simulink model "sudoku"  (R2012b)
settings: Solver=ode45  StartTime=0.0  StopTime=10.0  RelTol=1e-3
libraries: sldvlib x83
(part 3 of 4)

== system sudoku/bounds9 ==
  In1 : Inport
  Assumption : sldvlib/Objectives and Constraints/Assumption  enabled=on  customAVTBlockType=Assumption  intervals=true  initial=off  dispValues=on  outEnabled=on
      settings: AttributesFormatString=%<intervals>
  Logical Operator : Logic  AllPortsSameDT=off  OutDataTypeStr=boolean
  geq : RelationalOperator  Operator=<=  OutDataTypeStr=boolean
  lb : Constant  OutDataTypeStr=int8
  leq : RelationalOperator  Operator=<=  OutDataTypeStr=boolean
  ub : Constant  Value=9  OutDataTypeStr=int8
  wires:
  In1/1 -> geq/1, leq/2
  geq/1 -> Logical Operator/2
  ub/1 -> geq/2
  leq/1 -> Logical Operator/1
  Logical Operator/1 -> Assumption/1
  lb/1 -> leq/1

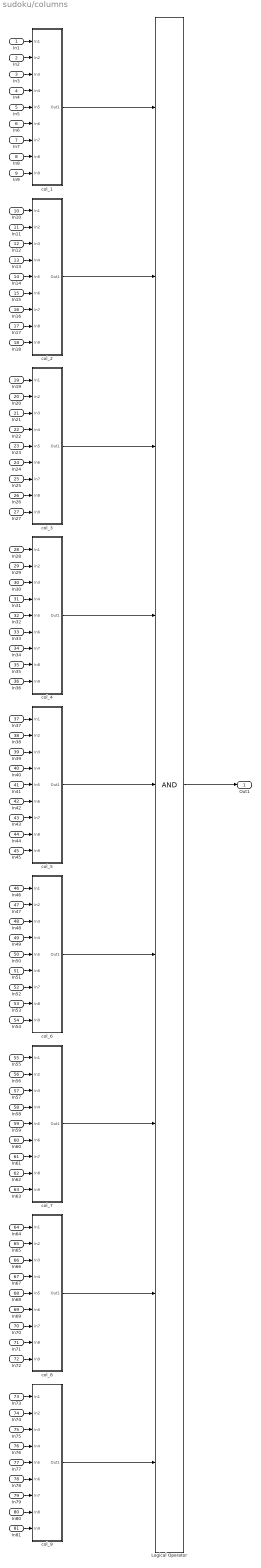
== system sudoku/columns ==
  In1 : Inport
  In2 : Inport  Port=2
  In3 : Inport  Port=3
  In4 : Inport  Port=4
  In5 : Inport  Port=5
  In6 : Inport  Port=6
  In7 : Inport  Port=7
  In8 : Inport  Port=8
  In9 : Inport  Port=9
  In10 : Inport  Port=10
  In11 : Inport  Port=11
  In12 : Inport  Port=12
  In13 : Inport  Port=13
  In14 : Inport  Port=14
  In15 : Inport  Port=15
  In16 : Inport  Port=16
  In17 : Inport  Port=17
  In18 : Inport  Port=18
  In19 : Inport  Port=19
  In20 : Inport  Port=20
  In21 : Inport  Port=21
  In22 : Inport  Port=22
  In23 : Inport  Port=23
  In24 : Inport  Port=24
  In25 : Inport  Port=25
  In26 : Inport  Port=26
  In27 : Inport  Port=27
  In28 : Inport  Port=28
  In29 : Inport  Port=29
  In30 : Inport  Port=30
  In31 : Inport  Port=31
  In32 : Inport  Port=32
  In33 : Inport  Port=33
  In34 : Inport  Port=34
  In35 : Inport  Port=35
  In36 : Inport  Port=36
  In37 : Inport  Port=37
  In38 : Inport  Port=38
  In39 : Inport  Port=39
  In40 : Inport  Port=40
  In41 : Inport  Port=41
  In42 : Inport  Port=42
  In43 : Inport  Port=43
  In44 : Inport  Port=44
  In45 : Inport  Port=45
  In46 : Inport  Port=46
  In47 : Inport  Port=47
  In48 : Inport  Port=48
  In49 : Inport  Port=49
  In50 : Inport  Port=50
  In51 : Inport  Port=51
  In52 : Inport  Port=52
  In53 : Inport  Port=53
  In54 : Inport  Port=54
  In55 : Inport  Port=55
  In56 : Inport  Port=56
  In57 : Inport  Port=57
  In58 : Inport  Port=58
  In59 : Inport  Port=59
  In60 : Inport  Port=60
  In61 : Inport  Port=61
  In62 : Inport  Port=62
  In63 : Inport  Port=63
  In64 : Inport  Port=64
  In65 : Inport  Port=65
  In66 : Inport  Port=66
  In67 : Inport  Port=67
  In68 : Inport  Port=68
  In69 : Inport  Port=69
  In70 : Inport  Port=70
  In71 : Inport  Port=71
  In72 : Inport  Port=72
  In73 : Inport  Port=73
  In74 : Inport  Port=74
  In75 : Inport  Port=75
  In76 : Inport  Port=76
  In77 : Inport  Port=77
  In78 : Inport  Port=78
  In79 : Inport  Port=79
  In80 : Inport  Port=80
  In81 : Inport  Port=81
  Logical Operator : Logic  Inputs=9  AllPortsSameDT=off  OutDataTypeStr=boolean
  col_1 : Subsystem
  col_2 : Subsystem
  col_3 : Subsystem
  col_4 : Subsystem
  col_5 : Subsystem
  col_6 : Subsystem
  col_7 : Subsystem
  col_8 : Subsystem
  col_9 : Subsystem
  Out1 : Outport
  wires:
  In13/1 -> col_2/4(In4)
  In10/1 -> col_2/1(In1)
  In14/1 -> col_2/5(In5)
  In16/1 -> col_2/7(In7)
  In18/1 -> col_2/9(In9)
  In12/1 -> col_2/3(In3)
  In63/1 -> col_7/9(In9)
  In62/1 -> col_7/8(In8)
  In17/1 -> col_2/8(In8)
  In11/1 -> col_2/2(In2)
  In15/1 -> col_2/6(In6)
  In47/1 -> col_6/2(In2)
  In48/1 -> col_6/3(In3)
  In59/1 -> col_7/5(In5)
  In60/1 -> col_7/6(In6)
  In56/1 -> col_7/2(In2)
  In57/1 -> col_7/3(In3)
  In58/1 -> col_7/4(In4)
  In55/1 -> col_7/1(In1)
  In61/1 -> col_7/7(In7)
  In32/1 -> col_4/5(In5)
  In33/1 -> col_4/6(In6)
  In28/1 -> col_4/1(In1)
  In2/1 -> col_1/2(In2)
  In4/1 -> col_1/4(In4)
  In8/1 -> col_1/8(In8)
  In9/1 -> col_1/9(In9)
  In35/1 -> col_4/8(In8)
  In34/1 -> col_4/7(In7)
  In1/1 -> col_1/1(In1)
  In6/1 -> col_1/6(In6)
  In7/1 -> col_1/7(In7)
  In49/1 -> col_6/4(In4)
  In50/1 -> col_6/5(In5)
  In51/1 -> col_6/6(In6)
  In52/1 -> col_6/7(In7)
  In53/1 -> col_6/8(In8)
  In3/1 -> col_1/3(In3)
  In54/1 -> col_6/9(In9)
  In37/1 -> col_5/1(In1)
  In46/1 -> col_6/1(In1)
  In5/1 -> col_1/5(In5)
  In38/1 -> col_5/2(In2)
  In39/1 -> col_5/3(In3)
  In36/1 -> col_4/9(In9)
  In29/1 -> col_4/2(In2)
  In30/1 -> col_4/3(In3)
  In31/1 -> col_4/4(In4)
  In65/1 -> col_8/2(In2)
  In43/1 -> col_5/7(In7)
  In72/1 -> col_8/9(In9)
  In69/1 -> col_8/6(In6)
  In20/1 -> col_3/2(In2)
  In25/1 -> col_3/7(In7)
  In80/1 -> col_9/8(In8)
  In42/1 -> col_5/6(In6)
  In22/1 -> col_3/4(In4)
  In45/1 -> col_5/9(In9)
  In71/1 -> col_8/8(In8)
  In79/1 -> col_9/7(In7)
  In26/1 -> col_3/8(In8)
  In76/1 -> col_9/4(In4)
  In77/1 -> col_9/5(In5)
  In21/1 -> col_3/3(In3)
  In67/1 -> col_8/4(In4)
  In68/1 -> col_8/5(In5)
  In75/1 -> col_9/3(In3)
  In64/1 -> col_8/1(In1)
  In27/1 -> col_3/9(In9)
  In81/1 -> col_9/9(In9)
  In70/1 -> col_8/7(In7)
  In23/1 -> col_3/5(In5)
  In73/1 -> col_9/1(In1)
  In41/1 -> col_5/5(In5)
  In24/1 -> col_3/6(In6)
  In44/1 -> col_5/8(In8)
  In74/1 -> col_9/2(In2)
  In40/1 -> col_5/4(In4)
  In66/1 -> col_8/3(In3)
  In78/1 -> col_9/6(In6)
  In19/1 -> col_3/1(In1)
  col_1/1(Out1) -> Logical Operator/1
  col_2/1(Out1) -> Logical Operator/2
  col_3/1(Out1) -> Logical Operator/3
  col_4/1(Out1) -> Logical Operator/4
  col_5/1(Out1) -> Logical Operator/5
  col_6/1(Out1) -> Logical Operator/6
  col_7/1(Out1) -> Logical Operator/7
  col_8/1(Out1) -> Logical Operator/8
  col_9/1(Out1) -> Logical Operator/9
  Logical Operator/1 -> Out1/1

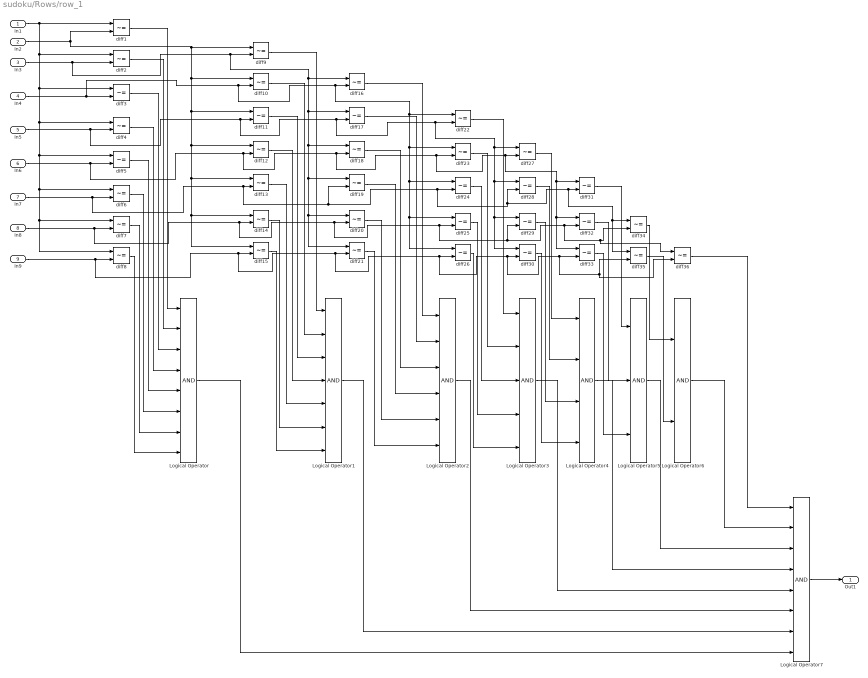
== system sudoku/Rows/row_1 ==
  In1 : Inport
  In2 : Inport  Port=2
  In3 : Inport  Port=3
  In4 : Inport  Port=4
  In5 : Inport  Port=5
  In6 : Inport  Port=6
  In7 : Inport  Port=7
  In8 : Inport  Port=8
  In9 : Inport  Port=9
  Logical Operator : Logic  Inputs=8  AllPortsSameDT=off  OutDataTypeStr=boolean
  Logical Operator1 : Logic  Inputs=7  AllPortsSameDT=off  OutDataTypeStr=boolean
  Logical Operator2 : Logic  Inputs=6  AllPortsSameDT=off  OutDataTypeStr=boolean
  Logical Operator3 : Logic  Inputs=5  AllPortsSameDT=off  OutDataTypeStr=boolean
  Logical Operator4 : Logic  Inputs=4  AllPortsSameDT=off  OutDataTypeStr=boolean
  Logical Operator5 : Logic  Inputs=3  AllPortsSameDT=off  OutDataTypeStr=boolean
  Logical Operator6 : Logic  AllPortsSameDT=off  OutDataTypeStr=boolean
  Logical Operator7 : Logic  Inputs=8  AllPortsSameDT=off  OutDataTypeStr=boolean
  diff{1..36} (36 alike) : RelationalOperator  Operator=~=  OutDataTypeStr=boolean
  Out1 : Outport
  wires:
  In2/1 -> diff1/2, diff15/1, diff14/1, diff13/1, diff12/1, diff11/1, diff10/1, diff9/1
  In1/1 -> diff8/1, diff7/1, diff6/1, diff5/1, diff4/1, diff3/1, diff2/1, diff1/1
  In5/1 -> diff30/1, diff29/1, diff28/1, diff27/1, diff22/2, diff17/2, diff11/2, diff4/2
  In6/1 -> diff33/1, diff32/1, diff31/1, diff27/2, diff23/2, diff18/2, diff12/2, diff5/2
  In7/1 -> diff19/2, diff35/1, diff34/1, diff31/2, diff28/2, diff24/2, diff13/2, diff6/2
  diff1/1 -> Logical Operator/1
  In3/1 -> diff2/2, diff21/1, diff20/1, diff19/1, diff18/1, diff17/1, diff16/1, diff9/2
  In4/1 -> diff26/1, diff25/1, diff24/1, diff23/1, diff22/1, diff16/2, diff10/2, diff3/2
  diff8/1 -> Logical Operator/8
  diff26/1 -> Logical Operator3/5
  diff36/1 -> Logical Operator7/1
  Logical Operator1/1 -> Logical Operator7/7
  diff10/1 -> Logical Operator1/2
  diff18/1 -> Logical Operator2/3
  diff17/1 -> Logical Operator2/2
  diff31/1 -> Logical Operator5/1
  Logical Operator5/1 -> Logical Operator7/3
  diff34/1 -> Logical Operator6/1
  diff16/1 -> Logical Operator2/1
  diff33/1 -> Logical Operator5/3
  diff22/1 -> Logical Operator3/1
  diff35/1 -> Logical Operator6/2
  diff27/1 -> Logical Operator4/1
  Logical Operator/1 -> Logical Operator7/8
  diff25/1 -> Logical Operator3/4
  diff3/1 -> Logical Operator/3
  diff2/1 -> Logical Operator/2
  diff7/1 -> Logical Operator/7
  diff5/1 -> Logical Operator/5
  diff4/1 -> Logical Operator/4
  diff30/1 -> Logical Operator4/4
  Logical Operator7/1 -> Out1/1
  Logical Operator3/1 -> Logical Operator7/5
  Logical Operator6/1 -> Logical Operator7/2
  diff14/1 -> Logical Operator1/6
  Logical Operator2/1 -> Logical Operator7/6
  diff15/1 -> Logical Operator1/7
  diff32/1 -> Logical Operator5/2
  diff21/1 -> Logical Operator2/6
  Logical Operator4/1 -> Logical Operator7/4
  diff19/1 -> Logical Operator2/4
  diff20/1 -> Logical Operator2/5
  diff28/1 -> Logical Operator4/2
  In8/1 -> diff29/2, diff36/1, diff34/2, diff32/2, diff25/2, diff20/2, diff14/2, diff7/2
  diff29/1 -> Logical Operator4/3
  diff6/1 -> Logical Operator/6
  diff9/1 -> Logical Operator1/1
  diff23/1 -> Logical Operator3/2
  diff13/1 -> Logical Operator1/5
  diff24/1 -> Logical Operator3/3
  diff11/1 -> Logical Operator1/3
  diff12/1 -> Logical Operator1/4
  In9/1 -> diff35/2, diff36/2, diff33/2, diff30/2, diff26/2, diff21/2, diff15/2, diff8/2

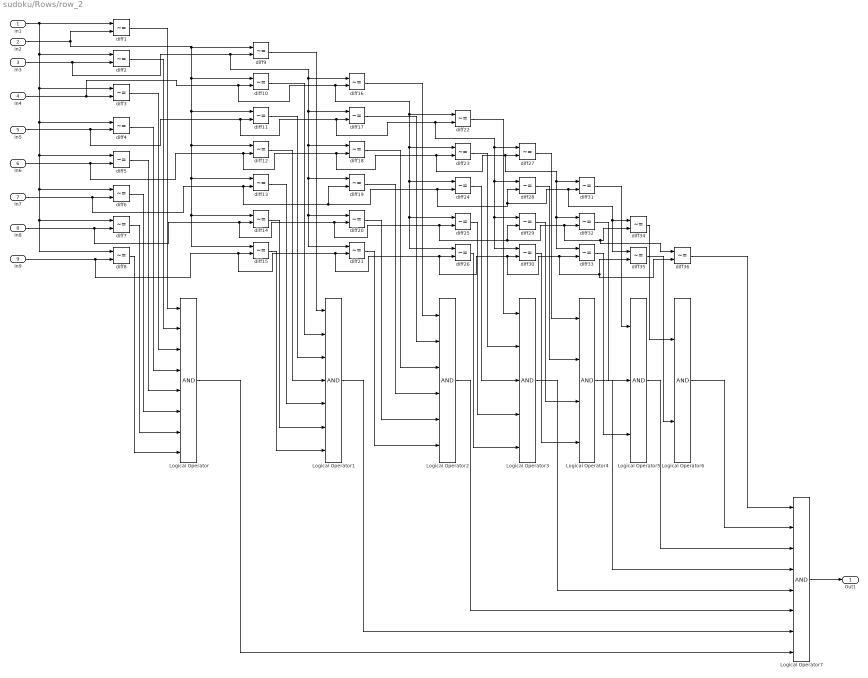
== system sudoku/Rows/row_2 ==
  In1 : Inport
  In2 : Inport  Port=2
  In3 : Inport  Port=3
  In4 : Inport  Port=4
  In5 : Inport  Port=5
  In6 : Inport  Port=6
  In7 : Inport  Port=7
  In8 : Inport  Port=8
  In9 : Inport  Port=9
  Logical Operator : Logic  Inputs=8  AllPortsSameDT=off  OutDataTypeStr=boolean
  Logical Operator1 : Logic  Inputs=7  AllPortsSameDT=off  OutDataTypeStr=boolean
  Logical Operator2 : Logic  Inputs=6  AllPortsSameDT=off  OutDataTypeStr=boolean
  Logical Operator3 : Logic  Inputs=5  AllPortsSameDT=off  OutDataTypeStr=boolean
  Logical Operator4 : Logic  Inputs=4  AllPortsSameDT=off  OutDataTypeStr=boolean
  Logical Operator5 : Logic  Inputs=3  AllPortsSameDT=off  OutDataTypeStr=boolean
  Logical Operator6 : Logic  AllPortsSameDT=off  OutDataTypeStr=boolean
  Logical Operator7 : Logic  Inputs=8  AllPortsSameDT=off  OutDataTypeStr=boolean
  diff{1..36} (36 alike) : RelationalOperator  Operator=~=  OutDataTypeStr=boolean
  Out1 : Outport
  wires:
  In2/1 -> diff1/2, diff15/1, diff14/1, diff13/1, diff12/1, diff11/1, diff10/1, diff9/1
  In1/1 -> diff8/1, diff7/1, diff6/1, diff5/1, diff4/1, diff3/1, diff2/1, diff1/1
  In5/1 -> diff30/1, diff29/1, diff28/1, diff27/1, diff22/2, diff17/2, diff11/2, diff4/2
  In6/1 -> diff33/1, diff32/1, diff31/1, diff27/2, diff23/2, diff18/2, diff12/2, diff5/2
  In7/1 -> diff19/2, diff35/1, diff34/1, diff31/2, diff28/2, diff24/2, diff13/2, diff6/2
  diff1/1 -> Logical Operator/1
  In3/1 -> diff2/2, diff21/1, diff20/1, diff19/1, diff18/1, diff17/1, diff16/1, diff9/2
  In4/1 -> diff26/1, diff25/1, diff24/1, diff23/1, diff22/1, diff16/2, diff10/2, diff3/2
  diff8/1 -> Logical Operator/8
  diff26/1 -> Logical Operator3/5
  diff36/1 -> Logical Operator7/1
  Logical Operator1/1 -> Logical Operator7/7
  diff10/1 -> Logical Operator1/2
  diff18/1 -> Logical Operator2/3
  diff17/1 -> Logical Operator2/2
  diff31/1 -> Logical Operator5/1
  Logical Operator5/1 -> Logical Operator7/3
  diff34/1 -> Logical Operator6/1
  diff16/1 -> Logical Operator2/1
  diff33/1 -> Logical Operator5/3
  diff22/1 -> Logical Operator3/1
  diff35/1 -> Logical Operator6/2
  diff27/1 -> Logical Operator4/1
  Logical Operator/1 -> Logical Operator7/8
  diff25/1 -> Logical Operator3/4
  diff3/1 -> Logical Operator/3
  diff2/1 -> Logical Operator/2
  diff7/1 -> Logical Operator/7
  diff5/1 -> Logical Operator/5
  diff4/1 -> Logical Operator/4
  diff30/1 -> Logical Operator4/4
  Logical Operator7/1 -> Out1/1
  Logical Operator3/1 -> Logical Operator7/5
  Logical Operator6/1 -> Logical Operator7/2
  diff14/1 -> Logical Operator1/6
  Logical Operator2/1 -> Logical Operator7/6
  diff15/1 -> Logical Operator1/7
  diff32/1 -> Logical Operator5/2
  diff21/1 -> Logical Operator2/6
  Logical Operator4/1 -> Logical Operator7/4
  diff19/1 -> Logical Operator2/4
  diff20/1 -> Logical Operator2/5
  diff28/1 -> Logical Operator4/2
  In8/1 -> diff29/2, diff36/1, diff34/2, diff32/2, diff25/2, diff20/2, diff14/2, diff7/2
  diff29/1 -> Logical Operator4/3
  diff6/1 -> Logical Operator/6
  diff9/1 -> Logical Operator1/1
  diff23/1 -> Logical Operator3/2
  diff13/1 -> Logical Operator1/5
  diff24/1 -> Logical Operator3/3
  diff11/1 -> Logical Operator1/3
  diff12/1 -> Logical Operator1/4
  In9/1 -> diff35/2, diff36/2, diff33/2, diff30/2, diff26/2, diff21/2, diff15/2, diff8/2

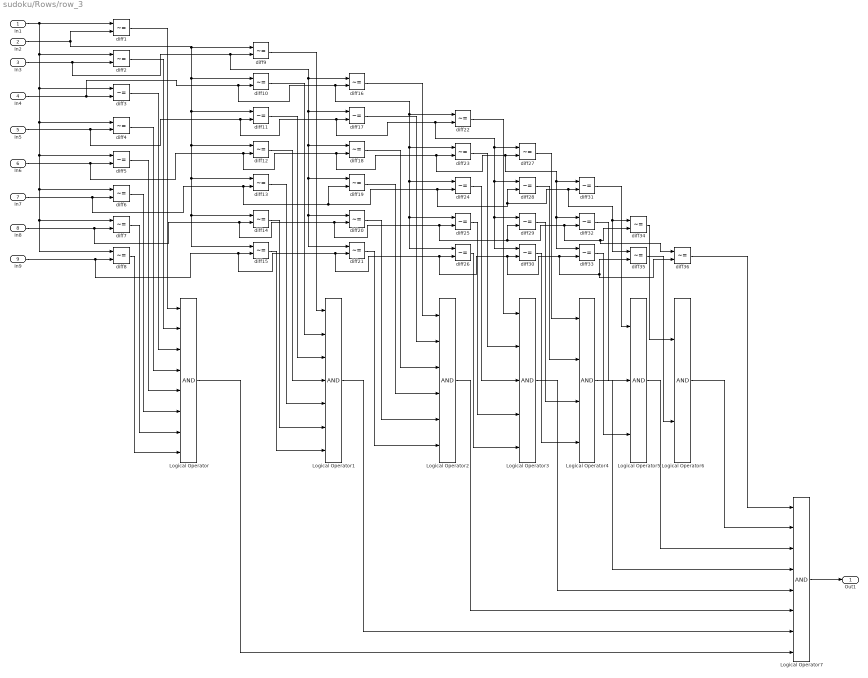
== system sudoku/Rows/row_3 ==
  In1 : Inport
  In2 : Inport  Port=2
  In3 : Inport  Port=3
  In4 : Inport  Port=4
  In5 : Inport  Port=5
  In6 : Inport  Port=6
  In7 : Inport  Port=7
  In8 : Inport  Port=8
  In9 : Inport  Port=9
  Logical Operator : Logic  Inputs=8  AllPortsSameDT=off  OutDataTypeStr=boolean
  Logical Operator1 : Logic  Inputs=7  AllPortsSameDT=off  OutDataTypeStr=boolean
  Logical Operator2 : Logic  Inputs=6  AllPortsSameDT=off  OutDataTypeStr=boolean
  Logical Operator3 : Logic  Inputs=5  AllPortsSameDT=off  OutDataTypeStr=boolean
  Logical Operator4 : Logic  Inputs=4  AllPortsSameDT=off  OutDataTypeStr=boolean
  Logical Operator5 : Logic  Inputs=3  AllPortsSameDT=off  OutDataTypeStr=boolean
  Logical Operator6 : Logic  AllPortsSameDT=off  OutDataTypeStr=boolean
  Logical Operator7 : Logic  Inputs=8  AllPortsSameDT=off  OutDataTypeStr=boolean
  diff{1..36} (36 alike) : RelationalOperator  Operator=~=  OutDataTypeStr=boolean
  Out1 : Outport
  wires:
  In2/1 -> diff1/2, diff15/1, diff14/1, diff13/1, diff12/1, diff11/1, diff10/1, diff9/1
  In1/1 -> diff8/1, diff7/1, diff6/1, diff5/1, diff4/1, diff3/1, diff2/1, diff1/1
  In5/1 -> diff30/1, diff29/1, diff28/1, diff27/1, diff22/2, diff17/2, diff11/2, diff4/2
  In6/1 -> diff33/1, diff32/1, diff31/1, diff27/2, diff23/2, diff18/2, diff12/2, diff5/2
  In7/1 -> diff19/2, diff35/1, diff34/1, diff31/2, diff28/2, diff24/2, diff13/2, diff6/2
  diff1/1 -> Logical Operator/1
  In3/1 -> diff2/2, diff21/1, diff20/1, diff19/1, diff18/1, diff17/1, diff16/1, diff9/2
  In4/1 -> diff26/1, diff25/1, diff24/1, diff23/1, diff22/1, diff16/2, diff10/2, diff3/2
  diff8/1 -> Logical Operator/8
  diff26/1 -> Logical Operator3/5
  diff36/1 -> Logical Operator7/1
  Logical Operator1/1 -> Logical Operator7/7
  diff10/1 -> Logical Operator1/2
  diff18/1 -> Logical Operator2/3
  diff17/1 -> Logical Operator2/2
  diff31/1 -> Logical Operator5/1
  Logical Operator5/1 -> Logical Operator7/3
  diff34/1 -> Logical Operator6/1
  diff16/1 -> Logical Operator2/1
  diff33/1 -> Logical Operator5/3
  diff22/1 -> Logical Operator3/1
  diff35/1 -> Logical Operator6/2
  diff27/1 -> Logical Operator4/1
  Logical Operator/1 -> Logical Operator7/8
  diff25/1 -> Logical Operator3/4
  diff3/1 -> Logical Operator/3
  diff2/1 -> Logical Operator/2
  diff7/1 -> Logical Operator/7
  diff5/1 -> Logical Operator/5
  diff4/1 -> Logical Operator/4
  diff30/1 -> Logical Operator4/4
  Logical Operator7/1 -> Out1/1
  Logical Operator3/1 -> Logical Operator7/5
  Logical Operator6/1 -> Logical Operator7/2
  diff14/1 -> Logical Operator1/6
  Logical Operator2/1 -> Logical Operator7/6
  diff15/1 -> Logical Operator1/7
  diff32/1 -> Logical Operator5/2
  diff21/1 -> Logical Operator2/6
  Logical Operator4/1 -> Logical Operator7/4
  diff19/1 -> Logical Operator2/4
  diff20/1 -> Logical Operator2/5
  diff28/1 -> Logical Operator4/2
  In8/1 -> diff29/2, diff36/1, diff34/2, diff32/2, diff25/2, diff20/2, diff14/2, diff7/2
  diff29/1 -> Logical Operator4/3
  diff6/1 -> Logical Operator/6
  diff9/1 -> Logical Operator1/1
  diff23/1 -> Logical Operator3/2
  diff13/1 -> Logical Operator1/5
  diff24/1 -> Logical Operator3/3
  diff11/1 -> Logical Operator1/3
  diff12/1 -> Logical Operator1/4
  In9/1 -> diff35/2, diff36/2, diff33/2, diff30/2, diff26/2, diff21/2, diff15/2, diff8/2

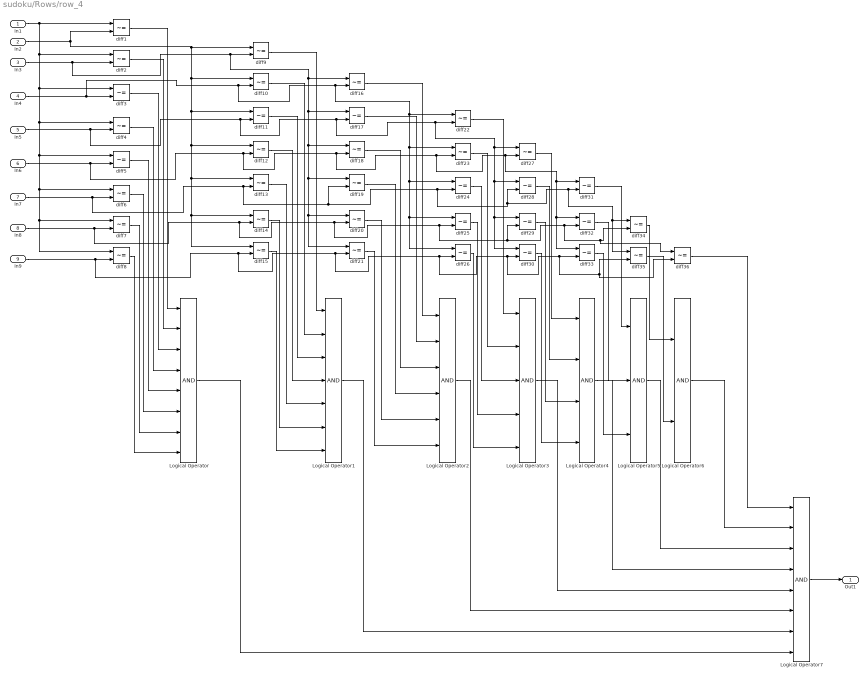
== system sudoku/Rows/row_4 ==
  In1 : Inport
  In2 : Inport  Port=2
  In3 : Inport  Port=3
  In4 : Inport  Port=4
  In5 : Inport  Port=5
  In6 : Inport  Port=6
  In7 : Inport  Port=7
  In8 : Inport  Port=8
  In9 : Inport  Port=9
  Logical Operator : Logic  Inputs=8  AllPortsSameDT=off  OutDataTypeStr=boolean
  Logical Operator1 : Logic  Inputs=7  AllPortsSameDT=off  OutDataTypeStr=boolean
  Logical Operator2 : Logic  Inputs=6  AllPortsSameDT=off  OutDataTypeStr=boolean
  Logical Operator3 : Logic  Inputs=5  AllPortsSameDT=off  OutDataTypeStr=boolean
  Logical Operator4 : Logic  Inputs=4  AllPortsSameDT=off  OutDataTypeStr=boolean
  Logical Operator5 : Logic  Inputs=3  AllPortsSameDT=off  OutDataTypeStr=boolean
  Logical Operator6 : Logic  AllPortsSameDT=off  OutDataTypeStr=boolean
  Logical Operator7 : Logic  Inputs=8  AllPortsSameDT=off  OutDataTypeStr=boolean
  diff{1..36} (36 alike) : RelationalOperator  Operator=~=  OutDataTypeStr=boolean
  Out1 : Outport
  wires:
  In2/1 -> diff1/2, diff15/1, diff14/1, diff13/1, diff12/1, diff11/1, diff10/1, diff9/1
  In1/1 -> diff8/1, diff7/1, diff6/1, diff5/1, diff4/1, diff3/1, diff2/1, diff1/1
  In5/1 -> diff30/1, diff29/1, diff28/1, diff27/1, diff22/2, diff17/2, diff11/2, diff4/2
  In6/1 -> diff33/1, diff32/1, diff31/1, diff27/2, diff23/2, diff18/2, diff12/2, diff5/2
  In7/1 -> diff19/2, diff35/1, diff34/1, diff31/2, diff28/2, diff24/2, diff13/2, diff6/2
  diff1/1 -> Logical Operator/1
  In3/1 -> diff2/2, diff21/1, diff20/1, diff19/1, diff18/1, diff17/1, diff16/1, diff9/2
  In4/1 -> diff26/1, diff25/1, diff24/1, diff23/1, diff22/1, diff16/2, diff10/2, diff3/2
  diff8/1 -> Logical Operator/8
  diff26/1 -> Logical Operator3/5
  diff36/1 -> Logical Operator7/1
  Logical Operator1/1 -> Logical Operator7/7
  diff10/1 -> Logical Operator1/2
  diff18/1 -> Logical Operator2/3
  diff17/1 -> Logical Operator2/2
  diff31/1 -> Logical Operator5/1
  Logical Operator5/1 -> Logical Operator7/3
  diff34/1 -> Logical Operator6/1
  diff16/1 -> Logical Operator2/1
  diff33/1 -> Logical Operator5/3
  diff22/1 -> Logical Operator3/1
  diff35/1 -> Logical Operator6/2
  diff27/1 -> Logical Operator4/1
  Logical Operator/1 -> Logical Operator7/8
  diff25/1 -> Logical Operator3/4
  diff3/1 -> Logical Operator/3
  diff2/1 -> Logical Operator/2
  diff7/1 -> Logical Operator/7
  diff5/1 -> Logical Operator/5
  diff4/1 -> Logical Operator/4
  diff30/1 -> Logical Operator4/4
  Logical Operator7/1 -> Out1/1
  Logical Operator3/1 -> Logical Operator7/5
  Logical Operator6/1 -> Logical Operator7/2
  diff14/1 -> Logical Operator1/6
  Logical Operator2/1 -> Logical Operator7/6
  diff15/1 -> Logical Operator1/7
  diff32/1 -> Logical Operator5/2
  diff21/1 -> Logical Operator2/6
  Logical Operator4/1 -> Logical Operator7/4
  diff19/1 -> Logical Operator2/4
  diff20/1 -> Logical Operator2/5
  diff28/1 -> Logical Operator4/2
  In8/1 -> diff29/2, diff36/1, diff34/2, diff32/2, diff25/2, diff20/2, diff14/2, diff7/2
  diff29/1 -> Logical Operator4/3
  diff6/1 -> Logical Operator/6
  diff9/1 -> Logical Operator1/1
  diff23/1 -> Logical Operator3/2
  diff13/1 -> Logical Operator1/5
  diff24/1 -> Logical Operator3/3
  diff11/1 -> Logical Operator1/3
  diff12/1 -> Logical Operator1/4
  In9/1 -> diff35/2, diff36/2, diff33/2, diff30/2, diff26/2, diff21/2, diff15/2, diff8/2

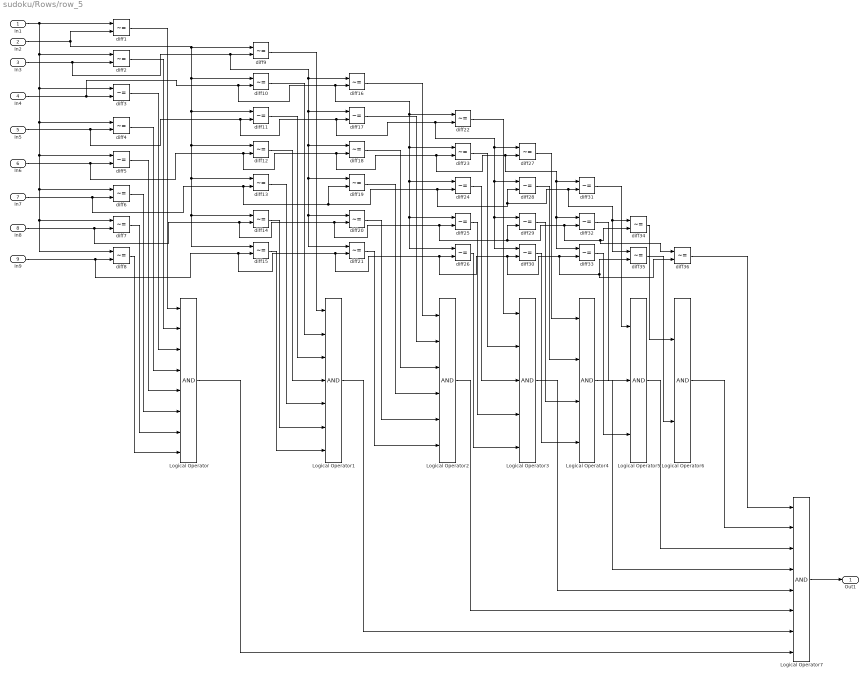
== system sudoku/Rows/row_5 ==
  In1 : Inport
  In2 : Inport  Port=2
  In3 : Inport  Port=3
  In4 : Inport  Port=4
  In5 : Inport  Port=5
  In6 : Inport  Port=6
  In7 : Inport  Port=7
  In8 : Inport  Port=8
  In9 : Inport  Port=9
  Logical Operator : Logic  Inputs=8  AllPortsSameDT=off  OutDataTypeStr=boolean
  Logical Operator1 : Logic  Inputs=7  AllPortsSameDT=off  OutDataTypeStr=boolean
  Logical Operator2 : Logic  Inputs=6  AllPortsSameDT=off  OutDataTypeStr=boolean
  Logical Operator3 : Logic  Inputs=5  AllPortsSameDT=off  OutDataTypeStr=boolean
  Logical Operator4 : Logic  Inputs=4  AllPortsSameDT=off  OutDataTypeStr=boolean
  Logical Operator5 : Logic  Inputs=3  AllPortsSameDT=off  OutDataTypeStr=boolean
  Logical Operator6 : Logic  AllPortsSameDT=off  OutDataTypeStr=boolean
  Logical Operator7 : Logic  Inputs=8  AllPortsSameDT=off  OutDataTypeStr=boolean
  diff{1..36} (36 alike) : RelationalOperator  Operator=~=  OutDataTypeStr=boolean
  Out1 : Outport
  wires:
  In2/1 -> diff1/2, diff15/1, diff14/1, diff13/1, diff12/1, diff11/1, diff10/1, diff9/1
  In1/1 -> diff8/1, diff7/1, diff6/1, diff5/1, diff4/1, diff3/1, diff2/1, diff1/1
  In5/1 -> diff30/1, diff29/1, diff28/1, diff27/1, diff22/2, diff17/2, diff11/2, diff4/2
  In6/1 -> diff33/1, diff32/1, diff31/1, diff27/2, diff23/2, diff18/2, diff12/2, diff5/2
  In7/1 -> diff19/2, diff35/1, diff34/1, diff31/2, diff28/2, diff24/2, diff13/2, diff6/2
  diff1/1 -> Logical Operator/1
  In3/1 -> diff2/2, diff21/1, diff20/1, diff19/1, diff18/1, diff17/1, diff16/1, diff9/2
  In4/1 -> diff26/1, diff25/1, diff24/1, diff23/1, diff22/1, diff16/2, diff10/2, diff3/2
  diff8/1 -> Logical Operator/8
  diff26/1 -> Logical Operator3/5
  diff36/1 -> Logical Operator7/1
  Logical Operator1/1 -> Logical Operator7/7
  diff10/1 -> Logical Operator1/2
  diff18/1 -> Logical Operator2/3
  diff17/1 -> Logical Operator2/2
  diff31/1 -> Logical Operator5/1
  Logical Operator5/1 -> Logical Operator7/3
  diff34/1 -> Logical Operator6/1
  diff16/1 -> Logical Operator2/1
  diff33/1 -> Logical Operator5/3
  diff22/1 -> Logical Operator3/1
  diff35/1 -> Logical Operator6/2
  diff27/1 -> Logical Operator4/1
  Logical Operator/1 -> Logical Operator7/8
  diff25/1 -> Logical Operator3/4
  diff3/1 -> Logical Operator/3
  diff2/1 -> Logical Operator/2
  diff7/1 -> Logical Operator/7
  diff5/1 -> Logical Operator/5
  diff4/1 -> Logical Operator/4
  diff30/1 -> Logical Operator4/4
  Logical Operator7/1 -> Out1/1
  Logical Operator3/1 -> Logical Operator7/5
  Logical Operator6/1 -> Logical Operator7/2
  diff14/1 -> Logical Operator1/6
  Logical Operator2/1 -> Logical Operator7/6
  diff15/1 -> Logical Operator1/7
  diff32/1 -> Logical Operator5/2
  diff21/1 -> Logical Operator2/6
  Logical Operator4/1 -> Logical Operator7/4
  diff19/1 -> Logical Operator2/4
  diff20/1 -> Logical Operator2/5
  diff28/1 -> Logical Operator4/2
  In8/1 -> diff29/2, diff36/1, diff34/2, diff32/2, diff25/2, diff20/2, diff14/2, diff7/2
  diff29/1 -> Logical Operator4/3
  diff6/1 -> Logical Operator/6
  diff9/1 -> Logical Operator1/1
  diff23/1 -> Logical Operator3/2
  diff13/1 -> Logical Operator1/5
  diff24/1 -> Logical Operator3/3
  diff11/1 -> Logical Operator1/3
  diff12/1 -> Logical Operator1/4
  In9/1 -> diff35/2, diff36/2, diff33/2, diff30/2, diff26/2, diff21/2, diff15/2, diff8/2

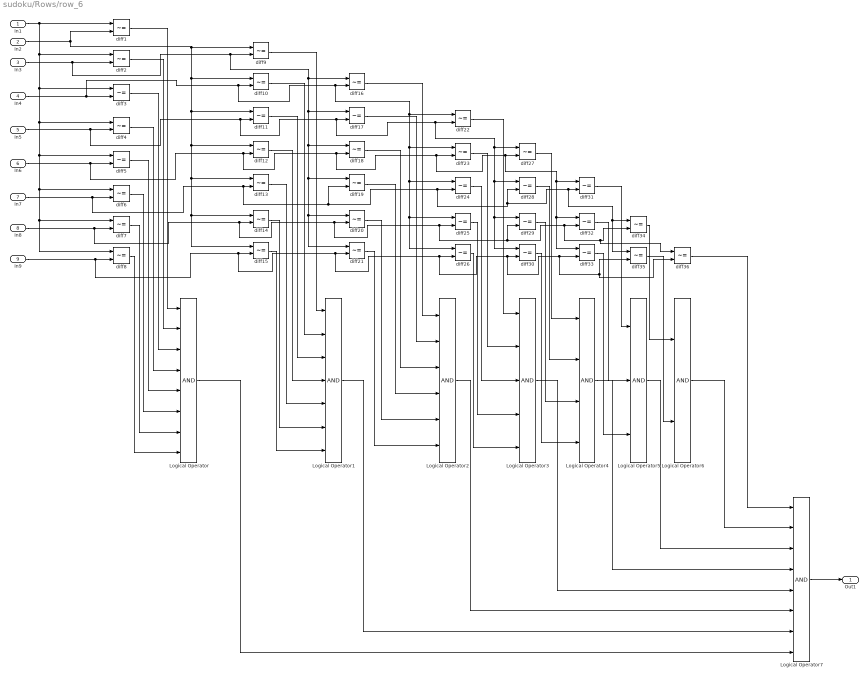
== system sudoku/Rows/row_6 ==
  In1 : Inport
  In2 : Inport  Port=2
  In3 : Inport  Port=3
  In4 : Inport  Port=4
  In5 : Inport  Port=5
  In6 : Inport  Port=6
  In7 : Inport  Port=7
  In8 : Inport  Port=8
  In9 : Inport  Port=9
  Logical Operator : Logic  Inputs=8  AllPortsSameDT=off  OutDataTypeStr=boolean
  Logical Operator1 : Logic  Inputs=7  AllPortsSameDT=off  OutDataTypeStr=boolean
  Logical Operator2 : Logic  Inputs=6  AllPortsSameDT=off  OutDataTypeStr=boolean
  Logical Operator3 : Logic  Inputs=5  AllPortsSameDT=off  OutDataTypeStr=boolean
  Logical Operator4 : Logic  Inputs=4  AllPortsSameDT=off  OutDataTypeStr=boolean
  Logical Operator5 : Logic  Inputs=3  AllPortsSameDT=off  OutDataTypeStr=boolean
  Logical Operator6 : Logic  AllPortsSameDT=off  OutDataTypeStr=boolean
  Logical Operator7 : Logic  Inputs=8  AllPortsSameDT=off  OutDataTypeStr=boolean
  diff{1..36} (36 alike) : RelationalOperator  Operator=~=  OutDataTypeStr=boolean
  Out1 : Outport
  wires:
  In2/1 -> diff1/2, diff15/1, diff14/1, diff13/1, diff12/1, diff11/1, diff10/1, diff9/1
  In1/1 -> diff8/1, diff7/1, diff6/1, diff5/1, diff4/1, diff3/1, diff2/1, diff1/1
  In5/1 -> diff30/1, diff29/1, diff28/1, diff27/1, diff22/2, diff17/2, diff11/2, diff4/2
  In6/1 -> diff33/1, diff32/1, diff31/1, diff27/2, diff23/2, diff18/2, diff12/2, diff5/2
  In7/1 -> diff19/2, diff35/1, diff34/1, diff31/2, diff28/2, diff24/2, diff13/2, diff6/2
  diff1/1 -> Logical Operator/1
  In3/1 -> diff2/2, diff21/1, diff20/1, diff19/1, diff18/1, diff17/1, diff16/1, diff9/2
  In4/1 -> diff26/1, diff25/1, diff24/1, diff23/1, diff22/1, diff16/2, diff10/2, diff3/2
  diff8/1 -> Logical Operator/8
  diff26/1 -> Logical Operator3/5
  diff36/1 -> Logical Operator7/1
  Logical Operator1/1 -> Logical Operator7/7
  diff10/1 -> Logical Operator1/2
  diff18/1 -> Logical Operator2/3
  diff17/1 -> Logical Operator2/2
  diff31/1 -> Logical Operator5/1
  Logical Operator5/1 -> Logical Operator7/3
  diff34/1 -> Logical Operator6/1
  diff16/1 -> Logical Operator2/1
  diff33/1 -> Logical Operator5/3
  diff22/1 -> Logical Operator3/1
  diff35/1 -> Logical Operator6/2
  diff27/1 -> Logical Operator4/1
  Logical Operator/1 -> Logical Operator7/8
  diff25/1 -> Logical Operator3/4
  diff3/1 -> Logical Operator/3
  diff2/1 -> Logical Operator/2
  diff7/1 -> Logical Operator/7
  diff5/1 -> Logical Operator/5
  diff4/1 -> Logical Operator/4
  diff30/1 -> Logical Operator4/4
  Logical Operator7/1 -> Out1/1
  Logical Operator3/1 -> Logical Operator7/5
  Logical Operator6/1 -> Logical Operator7/2
  diff14/1 -> Logical Operator1/6
  Logical Operator2/1 -> Logical Operator7/6
  diff15/1 -> Logical Operator1/7
  diff32/1 -> Logical Operator5/2
  diff21/1 -> Logical Operator2/6
  Logical Operator4/1 -> Logical Operator7/4
  diff19/1 -> Logical Operator2/4
  diff20/1 -> Logical Operator2/5
  diff28/1 -> Logical Operator4/2
  In8/1 -> diff29/2, diff36/1, diff34/2, diff32/2, diff25/2, diff20/2, diff14/2, diff7/2
  diff29/1 -> Logical Operator4/3
  diff6/1 -> Logical Operator/6
  diff9/1 -> Logical Operator1/1
  diff23/1 -> Logical Operator3/2
  diff13/1 -> Logical Operator1/5
  diff24/1 -> Logical Operator3/3
  diff11/1 -> Logical Operator1/3
  diff12/1 -> Logical Operator1/4
  In9/1 -> diff35/2, diff36/2, diff33/2, diff30/2, diff26/2, diff21/2, diff15/2, diff8/2

== system sudoku/Rows/row_7 ==
  In1 : Inport
  In2 : Inport  Port=2
  In3 : Inport  Port=3
  In4 : Inport  Port=4
  In5 : Inport  Port=5
  In6 : Inport  Port=6
  In7 : Inport  Port=7
  In8 : Inport  Port=8
  In9 : Inport  Port=9
  Logical Operator : Logic  Inputs=8  AllPortsSameDT=off  OutDataTypeStr=boolean
  Logical Operator1 : Logic  Inputs=7  AllPortsSameDT=off  OutDataTypeStr=boolean
  Logical Operator2 : Logic  Inputs=6  AllPortsSameDT=off  OutDataTypeStr=boolean
  Logical Operator3 : Logic  Inputs=5  AllPortsSameDT=off  OutDataTypeStr=boolean
  Logical Operator4 : Logic  Inputs=4  AllPortsSameDT=off  OutDataTypeStr=boolean
  Logical Operator5 : Logic  Inputs=3  AllPortsSameDT=off  OutDataTypeStr=boolean
  Logical Operator6 : Logic  AllPortsSameDT=off  OutDataTypeStr=boolean
  Logical Operator7 : Logic  Inputs=8  AllPortsSameDT=off  OutDataTypeStr=boolean
  diff{1..36} (36 alike) : RelationalOperator  Operator=~=  OutDataTypeStr=boolean
  Out1 : Outport
  wires:
  In2/1 -> diff1/2, diff15/1, diff14/1, diff13/1, diff12/1, diff11/1, diff10/1, diff9/1
  In1/1 -> diff8/1, diff7/1, diff6/1, diff5/1, diff4/1, diff3/1, diff2/1, diff1/1
  In5/1 -> diff30/1, diff29/1, diff28/1, diff27/1, diff22/2, diff17/2, diff11/2, diff4/2
  In6/1 -> diff33/1, diff32/1, diff31/1, diff27/2, diff23/2, diff18/2, diff12/2, diff5/2
  In7/1 -> diff19/2, diff35/1, diff34/1, diff31/2, diff28/2, diff24/2, diff13/2, diff6/2
  diff1/1 -> Logical Operator/1
  In3/1 -> diff2/2, diff21/1, diff20/1, diff19/1, diff18/1, diff17/1, diff16/1, diff9/2
  In4/1 -> diff26/1, diff25/1, diff24/1, diff23/1, diff22/1, diff16/2, diff10/2, diff3/2
  diff8/1 -> Logical Operator/8
  diff26/1 -> Logical Operator3/5
  diff36/1 -> Logical Operator7/1
  Logical Operator1/1 -> Logical Operator7/7
  diff10/1 -> Logical Operator1/2
  diff18/1 -> Logical Operator2/3
  diff17/1 -> Logical Operator2/2
  diff31/1 -> Logical Operator5/1
  Logical Operator5/1 -> Logical Operator7/3
  diff34/1 -> Logical Operator6/1
  diff16/1 -> Logical Operator2/1
  diff33/1 -> Logical Operator5/3
  diff22/1 -> Logical Operator3/1
  diff35/1 -> Logical Operator6/2
  diff27/1 -> Logical Operator4/1
  Logical Operator/1 -> Logical Operator7/8
  diff25/1 -> Logical Operator3/4
  diff3/1 -> Logical Operator/3
  diff2/1 -> Logical Operator/2
  diff7/1 -> Logical Operator/7
  diff5/1 -> Logical Operator/5
  diff4/1 -> Logical Operator/4
  diff30/1 -> Logical Operator4/4
  Logical Operator7/1 -> Out1/1
  Logical Operator3/1 -> Logical Operator7/5
  Logical Operator6/1 -> Logical Operator7/2
  diff14/1 -> Logical Operator1/6
  Logical Operator2/1 -> Logical Operator7/6
  diff15/1 -> Logical Operator1/7
  diff32/1 -> Logical Operator5/2
  diff21/1 -> Logical Operator2/6
  Logical Operator4/1 -> Logical Operator7/4
  diff19/1 -> Logical Operator2/4
  diff20/1 -> Logical Operator2/5
  diff28/1 -> Logical Operator4/2
  In8/1 -> diff29/2, diff36/1, diff34/2, diff32/2, diff25/2, diff20/2, diff14/2, diff7/2
  diff29/1 -> Logical Operator4/3
  diff6/1 -> Logical Operator/6
  diff9/1 -> Logical Operator1/1
  diff23/1 -> Logical Operator3/2
  diff13/1 -> Logical Operator1/5
  diff24/1 -> Logical Operator3/3
  diff11/1 -> Logical Operator1/3
  diff12/1 -> Logical Operator1/4
  In9/1 -> diff35/2, diff36/2, diff33/2, diff30/2, diff26/2, diff21/2, diff15/2, diff8/2

== system sudoku/Rows/row_8 ==
  In1 : Inport
  In2 : Inport  Port=2
  In3 : Inport  Port=3
  In4 : Inport  Port=4
  In5 : Inport  Port=5
  In6 : Inport  Port=6
  In7 : Inport  Port=7
  In8 : Inport  Port=8
  In9 : Inport  Port=9
  Logical Operator : Logic  Inputs=8  AllPortsSameDT=off  OutDataTypeStr=boolean
  Logical Operator1 : Logic  Inputs=7  AllPortsSameDT=off  OutDataTypeStr=boolean
  Logical Operator2 : Logic  Inputs=6  AllPortsSameDT=off  OutDataTypeStr=boolean
  Logical Operator3 : Logic  Inputs=5  AllPortsSameDT=off  OutDataTypeStr=boolean
  Logical Operator4 : Logic  Inputs=4  AllPortsSameDT=off  OutDataTypeStr=boolean
  Logical Operator5 : Logic  Inputs=3  AllPortsSameDT=off  OutDataTypeStr=boolean
  Logical Operator6 : Logic  AllPortsSameDT=off  OutDataTypeStr=boolean
  Logical Operator7 : Logic  Inputs=8  AllPortsSameDT=off  OutDataTypeStr=boolean
  diff{1..36} (36 alike) : RelationalOperator  Operator=~=  OutDataTypeStr=boolean
  Out1 : Outport
  wires:
  In2/1 -> diff1/2, diff15/1, diff14/1, diff13/1, diff12/1, diff11/1, diff10/1, diff9/1
  In1/1 -> diff8/1, diff7/1, diff6/1, diff5/1, diff4/1, diff3/1, diff2/1, diff1/1
  In5/1 -> diff30/1, diff29/1, diff28/1, diff27/1, diff22/2, diff17/2, diff11/2, diff4/2
  In6/1 -> diff33/1, diff32/1, diff31/1, diff27/2, diff23/2, diff18/2, diff12/2, diff5/2
  In7/1 -> diff19/2, diff35/1, diff34/1, diff31/2, diff28/2, diff24/2, diff13/2, diff6/2
  diff1/1 -> Logical Operator/1
  In3/1 -> diff2/2, diff21/1, diff20/1, diff19/1, diff18/1, diff17/1, diff16/1, diff9/2
  In4/1 -> diff26/1, diff25/1, diff24/1, diff23/1, diff22/1, diff16/2, diff10/2, diff3/2
  diff8/1 -> Logical Operator/8
  diff26/1 -> Logical Operator3/5
  diff36/1 -> Logical Operator7/1
  Logical Operator1/1 -> Logical Operator7/7
  diff10/1 -> Logical Operator1/2
  diff18/1 -> Logical Operator2/3
  diff17/1 -> Logical Operator2/2
  diff31/1 -> Logical Operator5/1
  Logical Operator5/1 -> Logical Operator7/3
  diff34/1 -> Logical Operator6/1
  diff16/1 -> Logical Operator2/1
  diff33/1 -> Logical Operator5/3
  diff22/1 -> Logical Operator3/1
  diff35/1 -> Logical Operator6/2
  diff27/1 -> Logical Operator4/1
  Logical Operator/1 -> Logical Operator7/8
  diff25/1 -> Logical Operator3/4
  diff3/1 -> Logical Operator/3
  diff2/1 -> Logical Operator/2
  diff7/1 -> Logical Operator/7
  diff5/1 -> Logical Operator/5
  diff4/1 -> Logical Operator/4
  diff30/1 -> Logical Operator4/4
  Logical Operator7/1 -> Out1/1
  Logical Operator3/1 -> Logical Operator7/5
  Logical Operator6/1 -> Logical Operator7/2
  diff14/1 -> Logical Operator1/6
  Logical Operator2/1 -> Logical Operator7/6
  diff15/1 -> Logical Operator1/7
  diff32/1 -> Logical Operator5/2
  diff21/1 -> Logical Operator2/6
  Logical Operator4/1 -> Logical Operator7/4
  diff19/1 -> Logical Operator2/4
  diff20/1 -> Logical Operator2/5
  diff28/1 -> Logical Operator4/2
  In8/1 -> diff29/2, diff36/1, diff34/2, diff32/2, diff25/2, diff20/2, diff14/2, diff7/2
  diff29/1 -> Logical Operator4/3
  diff6/1 -> Logical Operator/6
  diff9/1 -> Logical Operator1/1
  diff23/1 -> Logical Operator3/2
  diff13/1 -> Logical Operator1/5
  diff24/1 -> Logical Operator3/3
  diff11/1 -> Logical Operator1/3
  diff12/1 -> Logical Operator1/4
  In9/1 -> diff35/2, diff36/2, diff33/2, diff30/2, diff26/2, diff21/2, diff15/2, diff8/2

== system sudoku/Rows/row_9 ==
  In1 : Inport
  In2 : Inport  Port=2
  In3 : Inport  Port=3
  In4 : Inport  Port=4
  In5 : Inport  Port=5
  In6 : Inport  Port=6
  In7 : Inport  Port=7
  In8 : Inport  Port=8
  In9 : Inport  Port=9
  Logical Operator : Logic  Inputs=8  AllPortsSameDT=off  OutDataTypeStr=boolean
  Logical Operator1 : Logic  Inputs=7  AllPortsSameDT=off  OutDataTypeStr=boolean
  Logical Operator2 : Logic  Inputs=6  AllPortsSameDT=off  OutDataTypeStr=boolean
  Logical Operator3 : Logic  Inputs=5  AllPortsSameDT=off  OutDataTypeStr=boolean
  Logical Operator4 : Logic  Inputs=4  AllPortsSameDT=off  OutDataTypeStr=boolean
  Logical Operator5 : Logic  Inputs=3  AllPortsSameDT=off  OutDataTypeStr=boolean
  Logical Operator6 : Logic  AllPortsSameDT=off  OutDataTypeStr=boolean
  Logical Operator7 : Logic  Inputs=8  AllPortsSameDT=off  OutDataTypeStr=boolean
  diff{1..36} (36 alike) : RelationalOperator  Operator=~=  OutDataTypeStr=boolean
  Out1 : Outport
  wires:
  In2/1 -> diff1/2, diff15/1, diff14/1, diff13/1, diff12/1, diff11/1, diff10/1, diff9/1
  In1/1 -> diff8/1, diff7/1, diff6/1, diff5/1, diff4/1, diff3/1, diff2/1, diff1/1
  In5/1 -> diff30/1, diff29/1, diff28/1, diff27/1, diff22/2, diff17/2, diff11/2, diff4/2
  In6/1 -> diff33/1, diff32/1, diff31/1, diff27/2, diff23/2, diff18/2, diff12/2, diff5/2
  In7/1 -> diff19/2, diff35/1, diff34/1, diff31/2, diff28/2, diff24/2, diff13/2, diff6/2
  diff1/1 -> Logical Operator/1
  In3/1 -> diff2/2, diff21/1, diff20/1, diff19/1, diff18/1, diff17/1, diff16/1, diff9/2
  In4/1 -> diff26/1, diff25/1, diff24/1, diff23/1, diff22/1, diff16/2, diff10/2, diff3/2
  diff8/1 -> Logical Operator/8
  diff26/1 -> Logical Operator3/5
  diff36/1 -> Logical Operator7/1
  Logical Operator1/1 -> Logical Operator7/7
  diff10/1 -> Logical Operator1/2
  diff18/1 -> Logical Operator2/3
  diff17/1 -> Logical Operator2/2
  diff31/1 -> Logical Operator5/1
  Logical Operator5/1 -> Logical Operator7/3
  diff34/1 -> Logical Operator6/1
  diff16/1 -> Logical Operator2/1
  diff33/1 -> Logical Operator5/3
  diff22/1 -> Logical Operator3/1
  diff35/1 -> Logical Operator6/2
  diff27/1 -> Logical Operator4/1
  Logical Operator/1 -> Logical Operator7/8
  diff25/1 -> Logical Operator3/4
  diff3/1 -> Logical Operator/3
  diff2/1 -> Logical Operator/2
  diff7/1 -> Logical Operator/7
  diff5/1 -> Logical Operator/5
  diff4/1 -> Logical Operator/4
  diff30/1 -> Logical Operator4/4
  Logical Operator7/1 -> Out1/1
  Logical Operator3/1 -> Logical Operator7/5
  Logical Operator6/1 -> Logical Operator7/2
  diff14/1 -> Logical Operator1/6
  Logical Operator2/1 -> Logical Operator7/6
  diff15/1 -> Logical Operator1/7
  diff32/1 -> Logical Operator5/2
  diff21/1 -> Logical Operator2/6
  Logical Operator4/1 -> Logical Operator7/4
  diff19/1 -> Logical Operator2/4
  diff20/1 -> Logical Operator2/5
  diff28/1 -> Logical Operator4/2
  In8/1 -> diff29/2, diff36/1, diff34/2, diff32/2, diff25/2, diff20/2, diff14/2, diff7/2
  diff29/1 -> Logical Operator4/3
  diff6/1 -> Logical Operator/6
  diff9/1 -> Logical Operator1/1
  diff23/1 -> Logical Operator3/2
  diff13/1 -> Logical Operator1/5
  diff24/1 -> Logical Operator3/3
  diff11/1 -> Logical Operator1/3
  diff12/1 -> Logical Operator1/4
  In9/1 -> diff35/2, diff36/2, diff33/2, diff30/2, diff26/2, diff21/2, diff15/2, diff8/2

== system sudoku/blocks/block_1 ==
  In1 : Inport
  In2 : Inport  Port=2
  In3 : Inport  Port=3
  In4 : Inport  Port=4
  In5 : Inport  Port=5
  In6 : Inport  Port=6
  In7 : Inport  Port=7
  In8 : Inport  Port=8
  In9 : Inport  Port=9
  Logical Operator : Logic  Inputs=8  AllPortsSameDT=off  OutDataTypeStr=boolean
  Logical Operator1 : Logic  Inputs=7  AllPortsSameDT=off  OutDataTypeStr=boolean
  Logical Operator2 : Logic  Inputs=6  AllPortsSameDT=off  OutDataTypeStr=boolean
  Logical Operator3 : Logic  Inputs=5  AllPortsSameDT=off  OutDataTypeStr=boolean
  Logical Operator4 : Logic  Inputs=4  AllPortsSameDT=off  OutDataTypeStr=boolean
  Logical Operator5 : Logic  Inputs=3  AllPortsSameDT=off  OutDataTypeStr=boolean
  Logical Operator6 : Logic  AllPortsSameDT=off  OutDataTypeStr=boolean
  Logical Operator7 : Logic  Inputs=8  AllPortsSameDT=off  OutDataTypeStr=boolean
  diff{1..36} (36 alike) : RelationalOperator  Operator=~=  OutDataTypeStr=boolean
  Out1 : Outport
  wires:
  In2/1 -> diff1/2, diff15/1, diff14/1, diff13/1, diff12/1, diff11/1, diff10/1, diff9/1
  In1/1 -> diff8/1, diff7/1, diff6/1, diff5/1, diff4/1, diff3/1, diff2/1, diff1/1
  In5/1 -> diff30/1, diff29/1, diff28/1, diff27/1, diff22/2, diff17/2, diff11/2, diff4/2
  In6/1 -> diff33/1, diff32/1, diff31/1, diff27/2, diff23/2, diff18/2, diff12/2, diff5/2
  In7/1 -> diff19/2, diff35/1, diff34/1, diff31/2, diff28/2, diff24/2, diff13/2, diff6/2
  diff1/1 -> Logical Operator/1
  In3/1 -> diff2/2, diff21/1, diff20/1, diff19/1, diff18/1, diff17/1, diff16/1, diff9/2
  In4/1 -> diff26/1, diff25/1, diff24/1, diff23/1, diff22/1, diff16/2, diff10/2, diff3/2
  diff8/1 -> Logical Operator/8
  diff26/1 -> Logical Operator3/5
  diff36/1 -> Logical Operator7/1
  Logical Operator1/1 -> Logical Operator7/7
  diff10/1 -> Logical Operator1/2
  diff18/1 -> Logical Operator2/3
  diff17/1 -> Logical Operator2/2
  diff31/1 -> Logical Operator5/1
  Logical Operator5/1 -> Logical Operator7/3
  diff34/1 -> Logical Operator6/1
  diff16/1 -> Logical Operator2/1
  diff33/1 -> Logical Operator5/3
  diff22/1 -> Logical Operator3/1
  diff35/1 -> Logical Operator6/2
  diff27/1 -> Logical Operator4/1
  Logical Operator/1 -> Logical Operator7/8
  diff25/1 -> Logical Operator3/4
  diff3/1 -> Logical Operator/3
  diff2/1 -> Logical Operator/2
  diff7/1 -> Logical Operator/7
  diff5/1 -> Logical Operator/5
  diff4/1 -> Logical Operator/4
  diff30/1 -> Logical Operator4/4
  Logical Operator7/1 -> Out1/1
  Logical Operator3/1 -> Logical Operator7/5
  Logical Operator6/1 -> Logical Operator7/2
  diff14/1 -> Logical Operator1/6
  Logical Operator2/1 -> Logical Operator7/6
  diff15/1 -> Logical Operator1/7
  diff32/1 -> Logical Operator5/2
  diff21/1 -> Logical Operator2/6
  Logical Operator4/1 -> Logical Operator7/4
  diff19/1 -> Logical Operator2/4
  diff20/1 -> Logical Operator2/5
  diff28/1 -> Logical Operator4/2
  In8/1 -> diff29/2, diff36/1, diff34/2, diff32/2, diff25/2, diff20/2, diff14/2, diff7/2
  diff29/1 -> Logical Operator4/3
  diff6/1 -> Logical Operator/6
  diff9/1 -> Logical Operator1/1
  diff23/1 -> Logical Operator3/2
  diff13/1 -> Logical Operator1/5
  diff24/1 -> Logical Operator3/3
  diff11/1 -> Logical Operator1/3
  diff12/1 -> Logical Operator1/4
  In9/1 -> diff35/2, diff36/2, diff33/2, diff30/2, diff26/2, diff21/2, diff15/2, diff8/2

== system sudoku/blocks/block_2 ==
  In1 : Inport
  In2 : Inport  Port=2
  In3 : Inport  Port=3
  In4 : Inport  Port=4
  In5 : Inport  Port=5
  In6 : Inport  Port=6
  In7 : Inport  Port=7
  In8 : Inport  Port=8
  In9 : Inport  Port=9
  Logical Operator : Logic  Inputs=8  AllPortsSameDT=off  OutDataTypeStr=boolean
  Logical Operator1 : Logic  Inputs=7  AllPortsSameDT=off  OutDataTypeStr=boolean
  Logical Operator2 : Logic  Inputs=6  AllPortsSameDT=off  OutDataTypeStr=boolean
  Logical Operator3 : Logic  Inputs=5  AllPortsSameDT=off  OutDataTypeStr=boolean
  Logical Operator4 : Logic  Inputs=4  AllPortsSameDT=off  OutDataTypeStr=boolean
  Logical Operator5 : Logic  Inputs=3  AllPortsSameDT=off  OutDataTypeStr=boolean
  Logical Operator6 : Logic  AllPortsSameDT=off  OutDataTypeStr=boolean
  Logical Operator7 : Logic  Inputs=8  AllPortsSameDT=off  OutDataTypeStr=boolean
  diff{1..36} (36 alike) : RelationalOperator  Operator=~=  OutDataTypeStr=boolean
  Out1 : Outport
  wires:
  In2/1 -> diff1/2, diff15/1, diff14/1, diff13/1, diff12/1, diff11/1, diff10/1, diff9/1
  In1/1 -> diff8/1, diff7/1, diff6/1, diff5/1, diff4/1, diff3/1, diff2/1, diff1/1
  In5/1 -> diff30/1, diff29/1, diff28/1, diff27/1, diff22/2, diff17/2, diff11/2, diff4/2
  In6/1 -> diff33/1, diff32/1, diff31/1, diff27/2, diff23/2, diff18/2, diff12/2, diff5/2
  In7/1 -> diff19/2, diff35/1, diff34/1, diff31/2, diff28/2, diff24/2, diff13/2, diff6/2
  diff1/1 -> Logical Operator/1
  In3/1 -> diff2/2, diff21/1, diff20/1, diff19/1, diff18/1, diff17/1, diff16/1, diff9/2
  In4/1 -> diff26/1, diff25/1, diff24/1, diff23/1, diff22/1, diff16/2, diff10/2, diff3/2
  diff8/1 -> Logical Operator/8
  diff26/1 -> Logical Operator3/5
  diff36/1 -> Logical Operator7/1
  Logical Operator1/1 -> Logical Operator7/7
  diff10/1 -> Logical Operator1/2
  diff18/1 -> Logical Operator2/3
  diff17/1 -> Logical Operator2/2
  diff31/1 -> Logical Operator5/1
  Logical Operator5/1 -> Logical Operator7/3
  diff34/1 -> Logical Operator6/1
  diff16/1 -> Logical Operator2/1
  diff33/1 -> Logical Operator5/3
  diff22/1 -> Logical Operator3/1
  diff35/1 -> Logical Operator6/2
  diff27/1 -> Logical Operator4/1
  Logical Operator/1 -> Logical Operator7/8
  diff25/1 -> Logical Operator3/4
  diff3/1 -> Logical Operator/3
  diff2/1 -> Logical Operator/2
  diff7/1 -> Logical Operator/7
  diff5/1 -> Logical Operator/5
  diff4/1 -> Logical Operator/4
  diff30/1 -> Logical Operator4/4
  Logical Operator7/1 -> Out1/1
  Logical Operator3/1 -> Logical Operator7/5
  Logical Operator6/1 -> Logical Operator7/2
  diff14/1 -> Logical Operator1/6
  Logical Operator2/1 -> Logical Operator7/6
  diff15/1 -> Logical Operator1/7
  diff32/1 -> Logical Operator5/2
  diff21/1 -> Logical Operator2/6
  Logical Operator4/1 -> Logical Operator7/4
  diff19/1 -> Logical Operator2/4
  diff20/1 -> Logical Operator2/5
  diff28/1 -> Logical Operator4/2
  In8/1 -> diff29/2, diff36/1, diff34/2, diff32/2, diff25/2, diff20/2, diff14/2, diff7/2
  diff29/1 -> Logical Operator4/3
  diff6/1 -> Logical Operator/6
  diff9/1 -> Logical Operator1/1
  diff23/1 -> Logical Operator3/2
  diff13/1 -> Logical Operator1/5
  diff24/1 -> Logical Operator3/3
  diff11/1 -> Logical Operator1/3
  diff12/1 -> Logical Operator1/4
  In9/1 -> diff35/2, diff36/2, diff33/2, diff30/2, diff26/2, diff21/2, diff15/2, diff8/2

== system sudoku/blocks/block_3 ==
  In1 : Inport
  In2 : Inport  Port=2
  In3 : Inport  Port=3
  In4 : Inport  Port=4
  In5 : Inport  Port=5
  In6 : Inport  Port=6
  In7 : Inport  Port=7
  In8 : Inport  Port=8
  In9 : Inport  Port=9
  Logical Operator : Logic  Inputs=8  AllPortsSameDT=off  OutDataTypeStr=boolean
  Logical Operator1 : Logic  Inputs=7  AllPortsSameDT=off  OutDataTypeStr=boolean
  Logical Operator2 : Logic  Inputs=6  AllPortsSameDT=off  OutDataTypeStr=boolean
  Logical Operator3 : Logic  Inputs=5  AllPortsSameDT=off  OutDataTypeStr=boolean
  Logical Operator4 : Logic  Inputs=4  AllPortsSameDT=off  OutDataTypeStr=boolean
  Logical Operator5 : Logic  Inputs=3  AllPortsSameDT=off  OutDataTypeStr=boolean
  Logical Operator6 : Logic  AllPortsSameDT=off  OutDataTypeStr=boolean
  Logical Operator7 : Logic  Inputs=8  AllPortsSameDT=off  OutDataTypeStr=boolean
  diff{1..36} (36 alike) : RelationalOperator  Operator=~=  OutDataTypeStr=boolean
  Out1 : Outport
  wires:
  In2/1 -> diff1/2, diff15/1, diff14/1, diff13/1, diff12/1, diff11/1, diff10/1, diff9/1
  In1/1 -> diff8/1, diff7/1, diff6/1, diff5/1, diff4/1, diff3/1, diff2/1, diff1/1
  In5/1 -> diff30/1, diff29/1, diff28/1, diff27/1, diff22/2, diff17/2, diff11/2, diff4/2
  In6/1 -> diff33/1, diff32/1, diff31/1, diff27/2, diff23/2, diff18/2, diff12/2, diff5/2
  In7/1 -> diff19/2, diff35/1, diff34/1, diff31/2, diff28/2, diff24/2, diff13/2, diff6/2
  diff1/1 -> Logical Operator/1
  In3/1 -> diff2/2, diff21/1, diff20/1, diff19/1, diff18/1, diff17/1, diff16/1, diff9/2
  In4/1 -> diff26/1, diff25/1, diff24/1, diff23/1, diff22/1, diff16/2, diff10/2, diff3/2
  diff8/1 -> Logical Operator/8
  diff26/1 -> Logical Operator3/5
  diff36/1 -> Logical Operator7/1
  Logical Operator1/1 -> Logical Operator7/7
  diff10/1 -> Logical Operator1/2
  diff18/1 -> Logical Operator2/3
  diff17/1 -> Logical Operator2/2
  diff31/1 -> Logical Operator5/1
  Logical Operator5/1 -> Logical Operator7/3
  diff34/1 -> Logical Operator6/1
  diff16/1 -> Logical Operator2/1
  diff33/1 -> Logical Operator5/3
  diff22/1 -> Logical Operator3/1
  diff35/1 -> Logical Operator6/2
  diff27/1 -> Logical Operator4/1
  Logical Operator/1 -> Logical Operator7/8
  diff25/1 -> Logical Operator3/4
  diff3/1 -> Logical Operator/3
  diff2/1 -> Logical Operator/2
  diff7/1 -> Logical Operator/7
  diff5/1 -> Logical Operator/5
  diff4/1 -> Logical Operator/4
  diff30/1 -> Logical Operator4/4
  Logical Operator7/1 -> Out1/1
  Logical Operator3/1 -> Logical Operator7/5
  Logical Operator6/1 -> Logical Operator7/2
  diff14/1 -> Logical Operator1/6
  Logical Operator2/1 -> Logical Operator7/6
  diff15/1 -> Logical Operator1/7
  diff32/1 -> Logical Operator5/2
  diff21/1 -> Logical Operator2/6
  Logical Operator4/1 -> Logical Operator7/4
  diff19/1 -> Logical Operator2/4
  diff20/1 -> Logical Operator2/5
  diff28/1 -> Logical Operator4/2
  In8/1 -> diff29/2, diff36/1, diff34/2, diff32/2, diff25/2, diff20/2, diff14/2, diff7/2
  diff29/1 -> Logical Operator4/3
  diff6/1 -> Logical Operator/6
  diff9/1 -> Logical Operator1/1
  diff23/1 -> Logical Operator3/2
  diff13/1 -> Logical Operator1/5
  diff24/1 -> Logical Operator3/3
  diff11/1 -> Logical Operator1/3
  diff12/1 -> Logical Operator1/4
  In9/1 -> diff35/2, diff36/2, diff33/2, diff30/2, diff26/2, diff21/2, diff15/2, diff8/2

== system sudoku/blocks/block_4 ==
  In1 : Inport
  In2 : Inport  Port=2
  In3 : Inport  Port=3
  In4 : Inport  Port=4
  In5 : Inport  Port=5
  In6 : Inport  Port=6
  In7 : Inport  Port=7
  In8 : Inport  Port=8
  In9 : Inport  Port=9
  Logical Operator : Logic  Inputs=8  AllPortsSameDT=off  OutDataTypeStr=boolean
  Logical Operator1 : Logic  Inputs=7  AllPortsSameDT=off  OutDataTypeStr=boolean
  Logical Operator2 : Logic  Inputs=6  AllPortsSameDT=off  OutDataTypeStr=boolean
  Logical Operator3 : Logic  Inputs=5  AllPortsSameDT=off  OutDataTypeStr=boolean
  Logical Operator4 : Logic  Inputs=4  AllPortsSameDT=off  OutDataTypeStr=boolean
  Logical Operator5 : Logic  Inputs=3  AllPortsSameDT=off  OutDataTypeStr=boolean
  Logical Operator6 : Logic  AllPortsSameDT=off  OutDataTypeStr=boolean
  Logical Operator7 : Logic  Inputs=8  AllPortsSameDT=off  OutDataTypeStr=boolean
  diff{1..36} (36 alike) : RelationalOperator  Operator=~=  OutDataTypeStr=boolean
  Out1 : Outport
  wires:
  In2/1 -> diff1/2, diff15/1, diff14/1, diff13/1, diff12/1, diff11/1, diff10/1, diff9/1
  In1/1 -> diff8/1, diff7/1, diff6/1, diff5/1, diff4/1, diff3/1, diff2/1, diff1/1
  In5/1 -> diff30/1, diff29/1, diff28/1, diff27/1, diff22/2, diff17/2, diff11/2, diff4/2
  In6/1 -> diff33/1, diff32/1, diff31/1, diff27/2, diff23/2, diff18/2, diff12/2, diff5/2
  In7/1 -> diff19/2, diff35/1, diff34/1, diff31/2, diff28/2, diff24/2, diff13/2, diff6/2
  diff1/1 -> Logical Operator/1
  In3/1 -> diff2/2, diff21/1, diff20/1, diff19/1, diff18/1, diff17/1, diff16/1, diff9/2
  In4/1 -> diff26/1, diff25/1, diff24/1, diff23/1, diff22/1, diff16/2, diff10/2, diff3/2
  diff8/1 -> Logical Operator/8
  diff26/1 -> Logical Operator3/5
  diff36/1 -> Logical Operator7/1
  Logical Operator1/1 -> Logical Operator7/7
  diff10/1 -> Logical Operator1/2
  diff18/1 -> Logical Operator2/3
  diff17/1 -> Logical Operator2/2
  diff31/1 -> Logical Operator5/1
  Logical Operator5/1 -> Logical Operator7/3
  diff34/1 -> Logical Operator6/1
  diff16/1 -> Logical Operator2/1
  diff33/1 -> Logical Operator5/3
  diff22/1 -> Logical Operator3/1
  diff35/1 -> Logical Operator6/2
  diff27/1 -> Logical Operator4/1
  Logical Operator/1 -> Logical Operator7/8
  diff25/1 -> Logical Operator3/4
  diff3/1 -> Logical Operator/3
  diff2/1 -> Logical Operator/2
  diff7/1 -> Logical Operator/7
  diff5/1 -> Logical Operator/5
  diff4/1 -> Logical Operator/4
  diff30/1 -> Logical Operator4/4
  Logical Operator7/1 -> Out1/1
  Logical Operator3/1 -> Logical Operator7/5
  Logical Operator6/1 -> Logical Operator7/2
  diff14/1 -> Logical Operator1/6
  Logical Operator2/1 -> Logical Operator7/6
  diff15/1 -> Logical Operator1/7
  diff32/1 -> Logical Operator5/2
  diff21/1 -> Logical Operator2/6
  Logical Operator4/1 -> Logical Operator7/4
  diff19/1 -> Logical Operator2/4
  diff20/1 -> Logical Operator2/5
  diff28/1 -> Logical Operator4/2
  In8/1 -> diff29/2, diff36/1, diff34/2, diff32/2, diff25/2, diff20/2, diff14/2, diff7/2
  diff29/1 -> Logical Operator4/3
  diff6/1 -> Logical Operator/6
  diff9/1 -> Logical Operator1/1
  diff23/1 -> Logical Operator3/2
  diff13/1 -> Logical Operator1/5
  diff24/1 -> Logical Operator3/3
  diff11/1 -> Logical Operator1/3
  diff12/1 -> Logical Operator1/4
  In9/1 -> diff35/2, diff36/2, diff33/2, diff30/2, diff26/2, diff21/2, diff15/2, diff8/2
